simulink model "ss_kalmf2"  (R2022b)
settings: Solver=ode4  StartTime=0.0  StopTime=10.0  FixedStep=.002  RelTol=1e-3
values from neighbouring files (symbols this model uses):
  a = 2    [RunMeFirst.m]
  A = exp(-a*Ts)    [RunMeFirst.m]    (also in linsys1.m = -a)
  B = 1    [RunMeFirst.m]    (also in linsys1.m = b)
  C = 1    [RunMeFirst.m]    (also in linsys1.m)
  D = 0    [RunMeFirst.m]    (also in linsys1.m)
  Qd = Q * G^2 * 1/(2*a) * (1 - exp(-2*a*Ts))    [RunMeFirst.m]
  R = .2    (= 0.2)    [RunMeFirst.m]    (also in linsys1.m = 0.5)
  Ts = .05    (= 0.05)    [RunMeFirst.m]    (also in linsys1.m = 0.1)
  x_0 = 2    [RunMeFirst.m]
  xe_0 = 3    [RunMeFirst.m]
undefined symbols (not defined in the file or in its folder): Discrete, K, Time
libraries: simulink x1, ctrlSharedLib x1
settings Model: Creator=hp_desktop  LastModifiedBy=hp_desktop

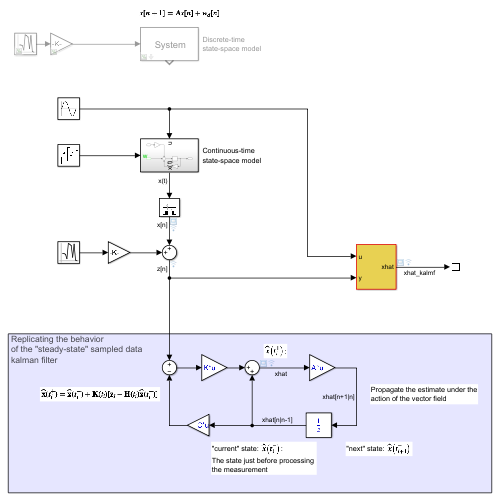
[thumbnail: Simulink's stored preview of the top-level diagram]
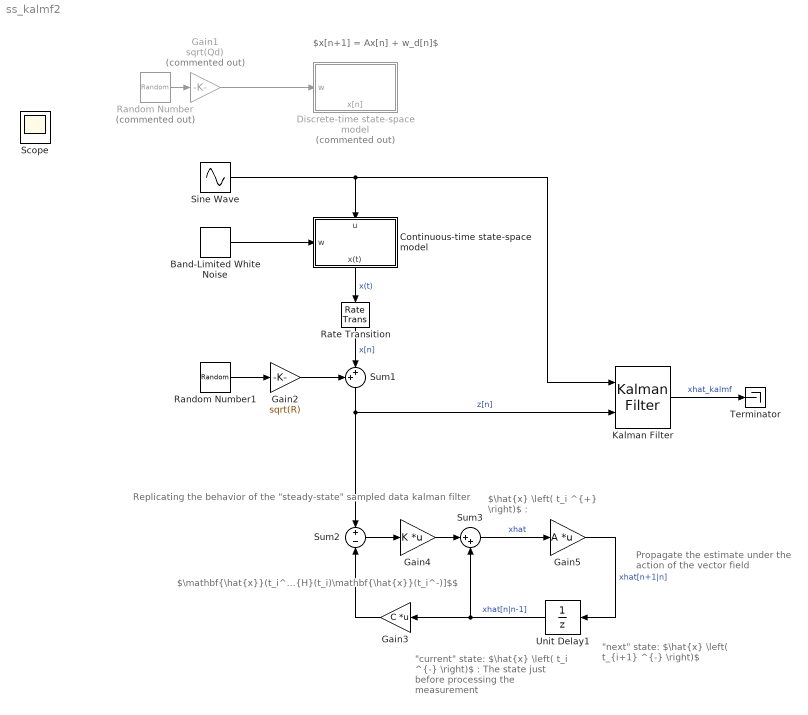
== system ss_kalmf2 ==
  note: Replicating the behavior
      | of the "steady-state" sampled data
      | kalman filter
  note: Propagate the estimate under the
      | action of the vector field
  note: $\mathbf{\hat{x}}(t_i^+)=\mathbf{\hat{x}}(t_i^-)+\mathbf{K}(t_i)[\mathbf{z}_i-\mathbf{H}(t_i)\mathbf{\hat{x}}(t_i^-)]$$
  note: "current" state: $\hat{x} \left( t_i ^{-} \right)$ :
      | The state just before processing
      | the measurement
  note: $x[n+1] = Ax[n] + w_d[n]$
  note: "next" state: $\hat{x} \left( t_{i+1} ^{-} \right)$
  note: $\hat{x} \left( t_i ^{+} \right)$ :
  Band-Limited White Noise : simulink/Sources/Band-Limited White Noise  Cov=Q  Ts=.01  seed=0
  Continuous-time state-space model : Subsystem
      settings: PortSchema="{\"entries\":[{\"content\":{\"sides\":[{\"content\":{\"connectorIds\":[\"In1\"]},\"type\":\"ConnectorPlacement.EquallySpacedRectSide\",\"uuid\":\"03aefd50-9202-4ba5-8d59-8bb562bb4022\"},{\"content\":{\"connectorIds\":[],\"side\":\"RIGHT\"},\"type\":\"ConnectorPlacement.EquallySpacedRectSide\",\"uuid\":\"1686d747-63e6-444b-902a-9e9b0bc573f1\"},{\"content\":{\"connectorIds\":[\"In2\"],\"side\":\"TOP\"},\"type\":\"ConnectorPlacement.EquallySpacedRectSide\",\"uuid\":\"82334134-1918-4078-909d-97976d506e34\"},{\"content\":{\"connectorIds\":[\"Out1\"],\"side\":\"BOTTOM\"},\"type\":\"ConnectorPlacement.EquallySpacedRectSide\",\"uuid\":\"6a42f511-d3ae-4f43-bbaf-a2320965212b\"}]},\"type\":\"ConnectorPlacement.EquallySpacedConnector\",\"uuid\":\"1127eaf5-13bd-4ad9-99ec-3bc039f81ae3\"}],\"packageUris\":[\"http://schema.mathworks.com/mf0/Connector/R2020b\"],\"version\":\"1.0\"}"
  Discrete-time state-space model : Subsystem  Commented=on
      settings: PortSchema="{\"entries\":[{\"content\":{\"sides\":[{\"content\":{\"connectorIds\":[\"In1\"]},\"type\":\"ConnectorPlacement.EquallySpacedRectSide\",\"uuid\":\"03aefd50-9202-4ba5-8d59-8bb562bb4022\"},{\"content\":{\"connectorIds\":[],\"side\":\"RIGHT\"},\"type\":\"ConnectorPlacement.EquallySpacedRectSide\",\"uuid\":\"1686d747-63e6-444b-902a-9e9b0bc573f1\"},{\"content\":{\"connectorIds\":[],\"side\":\"TOP\"},\"type\":\"ConnectorPlacement.EquallySpacedRectSide\",\"uuid\":\"82334134-1918-4078-909d-97976d506e34\"},{\"content\":{\"connectorIds\":[\"Out1\"],\"side\":\"BOTTOM\"},\"type\":\"ConnectorPlacement.EquallySpacedRectSide\",\"uuid\":\"6a42f511-d3ae-4f43-bbaf-a2320965212b\"}]},\"type\":\"ConnectorPlacement.EquallySpacedConnector\",\"uuid\":\"1127eaf5-13bd-4ad9-99ec-3bc039f81ae3\"}],\"packageUris\":[\"http://schema.mathworks.com/mf0/Connector/R2020b\"],\"version\":\"1.0\"}"
      mask Display: disp('\fontsize{13} System', 'texmode','on');
  Gain1 : Gain  Commented=on  Gain=sqrt(Qd)
  Gain2 : Gain  Gain=sqrt(R)
  Gain3 : Gain  Gain=C  Multiplication=Matrix(K*u)
  Gain4 : Gain  Gain=K  Multiplication=Matrix(K*u)
  Gain5 : Gain  Gain=A  Multiplication=Matrix(K*u)
  Kalman Filter : ctrlSharedLib/Kalman Filter  TimeDomain=Discrete-Time  UseCurrentEstimator=on  ModelSource=Individual A, B, C, D matrices  ModelSourceVariable=ss(0.95,1,1,0,1)  A=A  B=B  C=C  D=D  NumberOfStates=1  NumberOfInputs=1  NumberOfOutputs=1  InitialEstimateSource=Dialog  X0=xe_0  P0=10  UseK=off  UseGH=off  NumberOfProcessNoiseInputs=1  G=1  TimeInvariantG=on  H=0  TimeInvariantH=on  Q=Qd  TimeInvariantQ=on  R=R  TimeInvariantR=on  N=0  TimeInvariantN=on  AddInputPort=on  AddEnablePort=off  OutputEstimatedY=off  OutputP=off  Ts=Ts
  Random Number : RandomNumber  Commented=on  SampleTime=Ts
  Random Number1 : RandomNumber  Seed=1503  SampleTime=Ts
  Rate Transition : RateTransition  OutPortSampleTime=Ts
  Sine Wave : Sin  Amplitude=.5  SampleTime=0
  Sum1 : Sum  Inputs=++|
  Sum2 : Sum  Inputs=+-
  Sum3 : Sum  Inputs=|++
  Terminator : Terminator
  Unit Delay1 : UnitDelay  InitialCondition=xe_0  SampleTime=Ts  HasFrameUpgradeWarning=on
  Scope : Scope
  wires:
  Random Number/1 -> Gain1/1
  Random Number1/1 -> Gain2/1
  Gain2/1 -> Sum1/1
  Sum1/1 -> Kalman Filter/2, Sum2/1  "z[n]"
  Unit Delay1/1 -> Sum3/2, Gain3/1  "xhat[n|n-1]"
  Gain5/1 -> Unit Delay1/1  "xhat[n+1|n]"
  Gain3/1 -> Sum2/2
  Sum2/1 -> Gain4/1
  Gain4/1 -> Sum3/1
  Sum3/1 -> Gain5/1  "xhat"
  Sine Wave/1 -> Kalman Filter/1, Continuous-time state-space model/2(u)
  Kalman Filter/1 -> Terminator/1  "xhat_kalmf"
  Gain1/1 -> Discrete-time state-space model/1(w)
  Continuous-time state-space model/1(x(t)) -> Rate Transition/1  "x(t)"
  Band-Limited White Noise/1 -> Continuous-time state-space model/1(w)
  Rate Transition/1 -> Sum1/2  "x[n]"

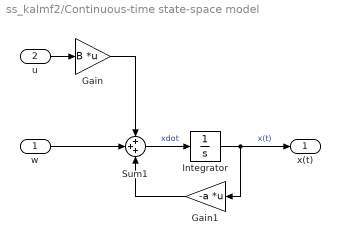
== system ss_kalmf2/Continuous-time state-space model ==
  w : Inport
  u : Inport  Port=2
  Gain : Gain  Gain=B  Multiplication=Matrix(K*u)
  Gain1 : Gain  Gain=-a  Multiplication=Matrix(K*u)
  Integrator : Integrator  InitialCondition=x_0
  Sum1 : Sum  Inputs=+++
  x(t) : Outport
  wires:
  Integrator/1 -> x(t)/1, Gain1/1  "x(t)"
  Sum1/1 -> Integrator/1  "xdot"
  Gain1/1 -> Sum1/3
  w/1 -> Sum1/2
  u/1 -> Gain/1
  Gain/1 -> Sum1/1

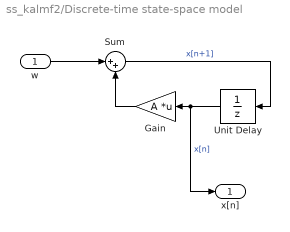
== system ss_kalmf2/Discrete-time state-space model ==
  w : Inport
  Gain : Gain  Gain=A  Multiplication=Matrix(K*u)
  Sum : Sum  Inputs=|++
  Unit Delay : UnitDelay  InitialCondition=x_0  SampleTime=-1  HasFrameUpgradeWarning=on
  x[n] : Outport
  wires:
  Unit Delay/1 -> x[n]/1, Gain/1  "x[n]"
  Gain/1 -> Sum/2
  Sum/1 -> Unit Delay/1  "x[n+1]"
  w/1 -> Sum/1
